simulink library "mec_pointmass_generic_ATvoith_DIWA_NXT"  (R2016a)
settings: Solver=ode45  SolverMode=SingleTasking  StartTime=0.0  StopTime=10.0  RelTol=1e-3
undefined symbols (not defined in the file): sMP
(part 1 of 4)
settings Model: Creator=pethama  LastModifiedBy=mhudelm
settings DataIOCC: LimitDataPoints=on  SaveFormat=Array
settings OptimizationCC: BlockReduction=off  BooleanDataType=off
settings DebuggingCC: SaveWithParameterizedLinksMsg=none  UnderspecifiedInitializationDetection=Classic  MergeDetectMultiDrivingBlocksExec=none  SignalResolutionControl=TryResolveAllWithWarning  StrictBusMsg=Warning
settings HardwareCC: ProdBitPerPointer=32  ProdLargestAtomicFloat=None  ProdIntDivRoundTo=Undefined  ProdEndianess=Unspecified  ProdWordSize=32  ProdHWDeviceType=32-bit Generic  TargetUnknown=on
settings ModelReferenceCC: PropagateSignalLabelsOutOfModel=off
settings ConfigComp: CovModelRefEnable=Off  CovSFcnEnable=off

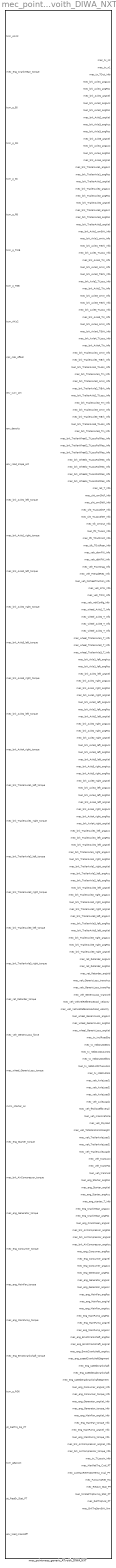
== system mec_pointmass_generic_ATvoith_DIWA_NXT ==
  "mec_pointmass_generic_ATvoith_DIWA_NXT " : Subsystem  mask{JCrankShaft_kgm2=sMP.phys.mec.eng.JCrankShaft_kgm2, JAirCompr=sMP.phys.mec.eng.JAirCompr, iAirCompr=sMP.phys.mec.eng.iAirCompr, airComprLoss_x_speed_rpm=sMP.phys.mec.eng.airComprLoss_x_speed_rpm, airComprLoss_map_lossTorque_Nm=sMP.phys.mec.eng.airComprLoss_map_lossTorque_Nm, JGenerator=sMP.phys.mec.mecConsumers.JGenerator, generatorLoss_x_speed_rpm=sMP.phys.mec.mecConsumers.generatorLoss_x_speed_rpm, generatorLoss_map_lossTorque_Nm=sMP.phys.mec.mecConsumers.generatorLoss_map_lossTorque_Nm, JEngConsumer=sMP.phys.mec.mecConsumers.JEngConsumer, engConsumerLoss_x_speed_rpm=sMP.phys.mec.mecConsumers.engConsumerLoss_x_speed_rpm, engConsumerLoss_y_torque_Nm=sMP.phys.mec.mecConsumers.engConsumerLoss_y_torque_Nm, engConsumerLoss_map_lossTorque_Nm=sMP.phys.mec.mecConsumers.engConsumerLoss_map_lossTorque_Nm, JMainFan=sMP.phys.mec.mecConsumers.JMainFan, mainFanLoss_x_speed_rpm=sMP.phys.mec.mecConsumers.mainFanLoss_x_speed_rpm, mainFanLoss_map_lossTorque_Nm=sMP.phys.mec.mecConsumers.mainFanLoss_map_lossTorque_Nm, JMainPump=sMP.phys.mec.mecConsumers.JMainPump, mainPumpLoss_x_speed_rpm=sMP.phys.mec.mecConsumers.mainPumpLoss_x_speed_rpm, mainPumpLoss_map_lossTorque_Nm=sMP.phys.mec.mecConsumers.mainPumpLoss_map_lossTorque_Nm, JEngEMot=sMP.phys.mec.mecConsumers.JEngEMot, engEMotLoss_x_speed_rpm=sMP.phys.mec.mecConsumers.engEMotLoss_x_speed_rpm, engEMotLoss_y_torque_Nm=sMP.phys.mec.mecConsumers.engEMotLoss_y_torque_Nm, engEMotLoss_map_lossTorque_Nm=sMP.phys.mec.mecConsumers.engEMotLoss_map_lossTorque_Nm, iStarter=sMP.phys.mec.eng.iStarter, scalAngVelStarter=sMP.phys.mec.eng.scalAngVelStarter}
      mask prompts: JCrankShaft_kgm2 "Inertia Crankshaft [kgm²]"; JAirCompr "Inertia AirCompressor [kgm²]"; iAirCompr "Ratio AirCompressor [-]"; airComprLoss_x_speed_rpm "Air Compressor Speed for Loss Torque Map [rpm]"; airComprLoss_map_lossTorque_Nm "Air Compressor Loss Torque Map [Nm]"; JGenerator "Inertia Generator [kgm²]"; generatorLoss_x_speed_rpm "Generator Speed for Loss Torque Map [rpm]"; generatorLoss_map_lossTorque_Nm "Generator Loss Torque Map [Nm]"; JEngConsumer "Inertia Generic Consumer Engine Crankshaft [kgm²]"; engConsumerLoss_x_speed_rpm "Generic Consumer Engine Crankshaft Speed for Loss Torque Map [rpm]"; engConsumerLoss_y_torque_Nm "Generic Consumer Engine Crankshaft Torque for Loss Torque Map [Nm]"; engConsumerLoss_map_lossTorque_Nm "Generic Consumer Engine Crankshaft Loss Torque Map [Nm]"; JMainFan "Inertia Main Fan [kgm²]"; mainFanLoss_x_speed_rpm "Main Fan Speed for Loss Torque Map [rpm]"; mainFanLoss_map_lossTorque_Nm "Main Fan Loss Torque Map [Nm]"; JMainPump "Inertia Main Pump [kgm²]"; mainPumpLoss_x_speed_rpm "Main Pump Speed for Loss Torque Map [rpm]"; mainPumpLoss_map_lossTorque_Nm "Main Pump Loss Torque Map [Nm]"; JEngEMot "Inertia E-Motor [kgm²]"; engEMotLoss_x_speed_rpm "E-Motor Engine Crankshaft Speed for Loss Torque Map [rpm]"; engEMotLoss_y_torque_Nm "E-Motor Engine Crankshaft Torque for Loss Torque Map [Nm]"; engEMotLoss_map_lossTorque_Nm "E-Motor Engine Crankshaft Loss Torque Map [Nm]"; iStarter "Ratio Starter [-]"; scalAngVelStarter "Scaling Factor for Angular Velocity  [-]"
